simulink subsystem "LowLevelController"  (R2023a)
settings: Solver=VariableStepAuto  StartTime=0.0  StopTime=10.0  RelTol=1e-3
model mask{K_m=16, K_cor=10}
  mask prompts: K_m "TorqueCoef, мН*м/А"; K_cor "PosledCorrect"
settings Model: Creator=pavelkuznecov  LastModifiedBy=agalimov

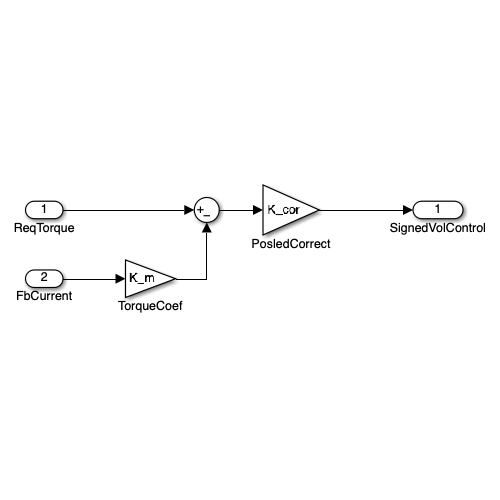
[thumbnail: Simulink's stored preview of the top-level diagram]
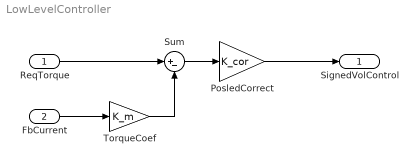
== system LowLevelController ==
  ReqTorque : Inport
  FbCurrent : Inport  Port=2
  PosledCorrect : Gain  Gain=K_cor
  Sum : Sum  Inputs=|+-
  TorqueCoef : Gain  Gain=K_m
  SignedVolControl : Outport
  wires:
  FbCurrent/1 -> TorqueCoef/1
  ReqTorque/1 -> Sum/1
  TorqueCoef/1 -> Sum/2
  Sum/1 -> PosledCorrect/1
  PosledCorrect/1 -> SignedVolControl/1
